simulink model "InputOutput"  (R2018b)
settings: Solver=VariableStepAuto  StartTime=0.0  StopTime=600  RelTol=1e-3
settings Model: Creator=danielazevedo  LastModifiedBy=Goncalopinto
settings SFSimCC: SimUseLocalCustomCode=off
settings RTWCC: RTWUseLocalCustomCode=off

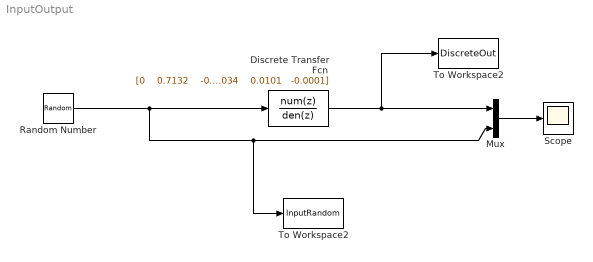
== system InputOutput ==
  Discrete Transfer Fcn : DiscreteTransferFcn  Numerator="[0    0.7132    -0.0323    -0.0087]"  Denominator="[1.0000   -0.2034    0.0101   -0.0001]"
  Mux : Mux  Inputs=2
  Random Number : RandomNumber  SampleTime=1
  Scope : Scope
  To Workspace2 : ToWorkspace  VariableName=DiscreteOut  SaveFormat=Timeseries  SampleTime=-1
  "To Workspace2 " : ToWorkspace  VariableName=InputRandom  SaveFormat=Timeseries  SampleTime=-1
  wires:
  Random Number/1 -> Mux/2, "To Workspace2 "/1, Discrete Transfer Fcn/1
  Discrete Transfer Fcn/1 -> To Workspace2/1, Mux/1
  Mux/1 -> Scope/1
